simulink model "MotMapped_EV_Front"  (R2020a)
settings: configuration reference "Reference" (kept outside this file)
undefined symbols (not defined in the file): w_eff_bp_EV_front
libraries: autolibmappedmotor x1
settings Model: DataDictionary=System_Data_Dictionary.sldd  ModifiedByFormat=The MathWorks, Inc.  PauseTimes=10  OrderedModelArguments=off  Creator=The MathWorks, Inc.  LastModifiedBy=The MathWorks, Inc.
settings ConfigSetRef: SourceName=Reference

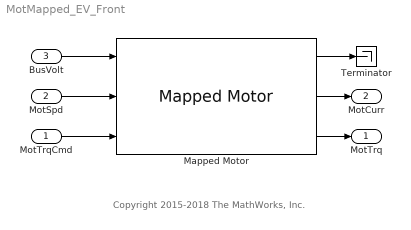
== system MotMapped_EV_Front ==
  note: Copyright 2015-2018 The MathWorks, Inc.
  MotTrqCmd : Inport
  MotSpd : Inport  Port=2
  BusVolt : Inport  Port=3
  Mapped Motor : autolibmappedmotor/Mapped Motor  port_config=Speed  param_by=Tabulated torque-speed envelope  w_t=w_eff_bp_EV_front.*pi/30  T_t=T_t_EV_front  torque_max=torque_max  power_max=power_max  Tc=Tc_Mot  param_loss=Tabulated efficiency data  eff=100  w_eff=375  T_eff=0.08  Piron=0  Pbase=0  w_eff_bp=w_eff_bp_EV_front.*pi/30  T_eff_bp=T_eff_bp_EV_front  Temp_eff_bp=[233.15 293.15 373.15]  losses_table=[1 2;3 4]  losses_table_3d=cat(3,1.05*[1.49 1.67 2.21 3.10; 0.42 0.69 1.14 2.03; 0.06 0.24 0.78 1.68; 0.42 0.69 1.14 2.03; 1.49 1.67 2.21 3.10],[1.49 1.67 2.21 3.10; 0.42 0.69 1.14 2.03; 0.06 0.24 0.78 1.68; 0.42 0.69 1.14 2.03; 1.49 1.67 2.21 3.10],1.03*[1.49 1.67 2.21 3.10; 0.42 0.69 1.14 2.03; 0.06 0.24 0.78 1.68; 0.42 0.69 1.14 2.03; 1.49 1.67 2.21 3.10])  efficiency_table=efficiency_table_EV  efficiency_table_3d=cat(3,90*ones(5,4),95*ones(5,4),92*ones(5,4))  J=5e-6  b=1e-5  omega_o=0  T_t_extended=[71.619724395 78.13060842 85.943669265 95.49296586 107.429586585 122.776670385 143.23944879 171.8873385 214.8591732 286.47889755 300 300 300 300 300 300 300 286.47889755 214.8591732 171.8873385 143.23944879 122.776670385 107.429586585 95.49296586 85.943669265 78.13060842 71.619724395]  w_t_extended=[-2094.3951023932 -1919.86217719376 -1745.32925199433 -1570.7963267949 -1396.26340159546 -1221.73047639603 -1047.1975511966 -872.664625997165 -698.131700797732 -523.598775598299 -499.998830689769 -349.065850398866 -174.532925199433 0 174.532925199433 349.065850398866 499.998830689769 523.598775598299 698.131700797732 872.664625997165 1047.1975511966 1221.73047639603 1396.26340159546 1570.7963267949 1745.32925199433 1919.86217719376 2094.3951023932]  KLossIron=0  KLossCopper=0  x_w_eff_vec=[-2094.3951023932 -1919.86217719376 -1745.32925199433 -1570.7963267949 -1396.26340159546 -1221.73047639603 -1047.1975511966 -872.664625997165 -698.131700797732 -523.598775598299 -499.998830689769 -349.065850398866 -174.532925199433 0 174.532925199433 349.065850398866 499.998830689769 523.598775598299 698.131700797732 872.664625997165 1047.1975511966 1221.73047639603 1396.26340159546 1570.7963267949 1745.32925199433 1919.86217719376 2094.3951023932]  x_T_eff_vec=[-300 -270 -240 -210 -180 -150 -120 -90 -60 -30 0 30 60 90 120 150 180 210 240 270 300]  x_tmp_eff_vec=[233.15 293.15 373.15]  x_losses_mat=[47292.792634685 42563.5133712165 37834.234107748 33104.9548442795 28375.675580811 23646.3963173425 18917.117053874 16390.9181926424 13962.6340159546 11087.9740714934 0 9424.77796076938 12566.3706143592 15079.644737231 17592.9188601028 21991.1485751285 26389.3782901542 30787.60800518 35185.8377202057 39584.0674352314 43982.2971502571;43351.7265817946 39016.5539236151 34681.3812654357 30346.2086072562 26011.0359490768 21675.8632908973 17340.6906327178 15025.0083432555 12799.0811812918 10163.9762322023 0 8639.37979737193 11519.1730631626 13823.0076757951 16126.8422884276 20158.5528605345 24190.2634326414 28221.9740047483 32253.6845768552 36285.3951489621 40317.105721069;39410.6605289042 35469.5944760138 31528.5284231233 27587.4623702329 23646.3963173425 19705.3302644521 15764.2642115617 13659.0984938687 11635.5283466289 9239.97839291116 0 7853.98163397448 10471.975511966 12566.3706143592 14660.7657167524 18325.9571459404 21991.1485751285 25656.3400043166 29321.5314335047 32986.7228626928 36651.9142918809;35469.5944760138 31922.6350284124 28375.675580811 24828.7161332096 21281.7566856083 17734.7972380069 14187.8377904055 12293.1886444818 10471.975511966 8315.98055362004 0 7068.58347057704 9424.77796076938 11309.7335529232 13194.6891450771 16493.3614313464 19792.0337176157 23090.706003885 26389.3782901542 29688.0505764235 32986.7228626928;26736.9587539557 24063.2628785601 21389.5670031645 18715.871127769 16042.1752523734 13368.4793769778 10694.7835015823 8021.0876261867 6305.70568462467 7391.98271432893 0 6283.18530717959 5864.30628670094 7539.8223686155 10053.0964914873 12566.3706143592 15079.644737231 17592.9188601028 20106.1929829747 22619.4671058465 25132.7412287183;19290.4812062531 17361.4330856278 15432.3849650025 13503.3368443772 11574.2887237519 9645.24060312655 7716.19248250124 7018.45167291337 5517.49247404658 6467.98487503781 0 5497.78714378214 5131.26800086332 6597.34457253856 7330.38285837617 9162.97857297022 10995.5742875643 12828.1700021583 14660.7657167523 16493.3614313464 18325.9571459404;16534.6981767884 14881.2283591095 13227.7585414307 11574.2887237519 9920.81890607302 8267.34908839418 6613.87927071535 6015.81571964003 4729.2792634685 5543.9870357467 0 4712.38898038469 4398.22971502571 5654.86677646162 6283.18530717958 7853.98163397447 9424.77796076937 10995.5742875643 12566.3706143592 14137.1669411541 15707.9632679489;13778.9151473236 12401.0236325913 11023.1321178589 9645.24060312655 8267.34908839418 6889.45757366182 6684.23968848892 5013.17976636669 3941.06605289042 4619.98919645558 0 3926.99081698724 3665.19142918809 4712.38898038469 6283.18530717958 6544.98469497873 7853.98163397447 9162.97857297022 10471.975511966 11780.9724509617 13089.9693899575;11023.1321178589 9920.81890607302 8818.50569428713 7716.19248250124 6613.87927071535 5511.56605892946 5347.39175079114 4010.54381309335 3152.85284231233 3695.99135716446 0 3141.59265358979 2932.15314335047 3769.91118430775 5026.54824574366 5235.98775598298 6283.18530717958 7330.38285837618 8377.58040957277 9424.77796076937 10471.975511966;10026.3595327334 9023.72357946004 8021.0876261867 7018.45167291337 6015.81571964003 5013.17976636669 4010.54381309335 3007.90785982001 2364.63963173425 2771.99351787335 0 2356.19449019235 2199.11485751285 2827.43338823081 3769.91118430775 4712.38898038469 5654.86677646162 6597.34457253856 7539.8223686155 8482.30016469243 9424.77796076937;13043.4477571244 11739.102981412 10434.7582056995 7903.20732380602 6774.17770611945 5645.14808843287 4516.1184707463 3913.03432713732 2608.68955142488 2647.05263306348 0 2249.99473810396 2399.99438731089 3599.99158096634 4199.99017779406 5249.98772224257 6299.98526669109 7349.9828111396 9599.97754924356 10799.974742899 11999.9719365545;9106.06566257911 8195.45909632119 7284.85253006328 6374.24596380537 5463.63939754746 4553.03283128955 3642.42626503164 2731.81969877373 1821.21313251582 1847.99567858223 0 1570.7963267949 1675.51608191456 2513.27412287183 3351.03216382911 4188.79020478639 ...(+4880 chars)]  x_losses_mat_3d=cat(3,[3.255 2.3205 1.7535 1.5645 1.7535 2.3205 3.255;2.1315 1.197 0.7245 0.441 0.7245 1.197 2.1315;1.764 0.819 0.252 0.063 0.252 0.819 1.764;2.1315 1.197 0.7245 0.441 0.7245 1.197 2.1315;3.255 2.3205 1.7535 1.5645 1.7535 2.3205 3.255],[3.1 2.21 1.67 1.49 1.67 2.21 3.1;2.03 1.14 0.69 0.42 0.69 1.14 2.03;1.68 0.78 0.24 0.06 0.24 0.78 1.68;2.03 1.14 0.69 0.42 0.69 1.14 2.03;3.1 2.21 1.67 1.49 1.67 2.21 3.1],[3.193 2.2763 1.7201 1.5347 1.7201 2.2763 3.193;2.0909 1.1742 0.7107 0.4326 0.7107 1.1742 2.0909;1.7304 0.8034 0.2472 0.0618 0.2472 0.8034 1.7304;2.0909 1.1742 0.7107 0.4326 0.7107 1.1742 2.0909;3.193 2.2763 1.7201 1.5347 1.7201 2.2763 3.193])  CalLossMapData={}  CalLossWithTempMapData={}  aMode=aMode  RefBlkName='autolibmappedmotor/Mapped Motor'
      settings: SourceProductBaseCode=PW,MT,VE,VP
  Terminator : Terminator
  MotTrq : Outport  VectorParamsAs1DForOutWhenUnconnected=off
  MotCurr : Outport  Port=2  VectorParamsAs1DForOutWhenUnconnected=off
  wires:
  MotTrqCmd/1 -> Mapped Motor/3
  BusVolt/1 -> Mapped Motor/1
  MotSpd/1 -> Mapped Motor/2
  Mapped Motor/3 -> MotTrq/1
  Mapped Motor/2 -> MotCurr/1
  Mapped Motor/1 -> Terminator/1
